simulink model "simple_FXTESO_ANSFT"  (R2024b)
settings: Solver=ode4  StartTime=0.0  StopTime=10  FixedStep=0.01  RelTol=1e-3
model workspace (MAT data in the model file):
  tra1 = [0 2 0 -2 0 2]
  tra2 = [0 2 2 2 2 0]
  tra3 = [0 0 2 2 2 2]
values from neighbouring files (symbols this model uses):
  F = 5    [assignment3.m]
undefined symbols (not defined in the file or in its folder): Light, MIL
libraries: dspobslib x7, simulink x3, robotcorelib x1, aerolibwind2 x1
settings Model: Creator=Adan Daniel  LastModifiedBy=danyy
settings OptimizationCC: ReuseModelBlockBuffer=off
settings RTWCC: GPUComputeCapability=3.5

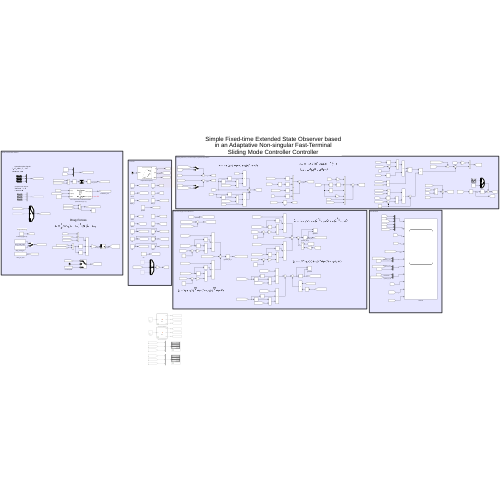
[thumbnail: Simulink's stored preview of the top-level diagram]
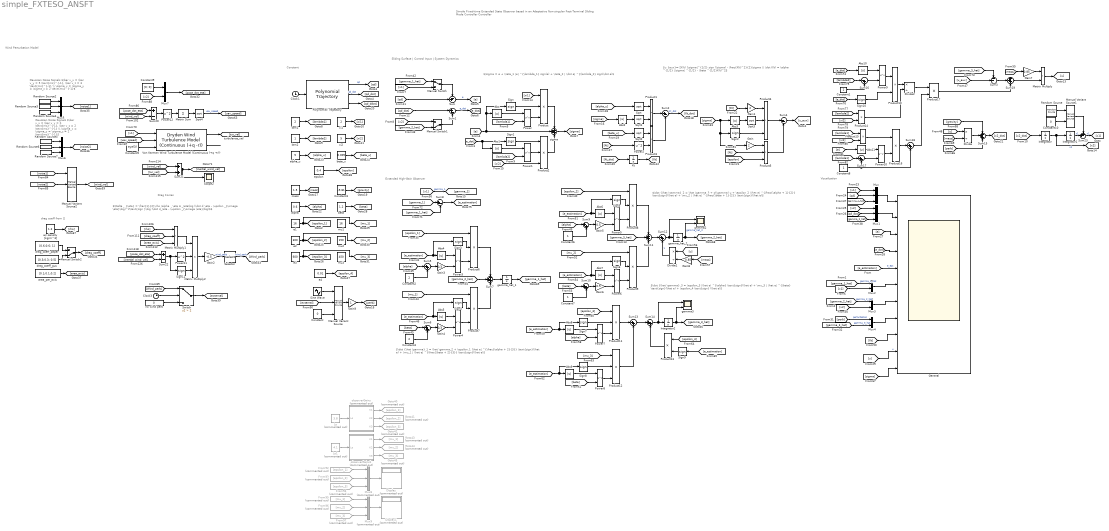
== system simple_FXTESO_ANSFT ==
  note: Extended High-Gain Observer
  note: Sliding Surface | Control Input | System Dynamics
  note: Constant
  note: Visualization
  note: Simple Fixed-time Extended State Observer based in an Adaptative Non-singular Fast-Terminal Sliding Mode Controller Controller
  note: $\dot {\hat \gamma}_1 = \hat \gamma_2 + \epsilon_1 |\hat e| ^{\frac{\alpha + 2}{3}} \text{sign}(\hat e) + \mu_1 | \hat e| ^{\frac{\beta + 2}{3}} \text{sign}(\hat e)$
  note: $\dot {\hat \gamma}_3 = \epsilon_3 |\hat e| ^{\alpha} \text{sign}(\hat e) + \mu_3 | \hat e| ^{\beta} \text{sign}(\hat e) + \epsilon_4 \text{sign} (\hat e)$
  note: $\dot {\hat \gamma}_2 = \hat \gamma_3 + g(\gamma) u + \epsilon_2 |\hat e| ^{\frac{\alpha + 1}{2}} \text{sign}(\hat e) + \mu_2 | \hat e| ^{\frac{\beta + 1}{2}} \text{sign}(\hat e)$
  note: $\sigma = e + \zeta_1 |e| ^{\lambda_1} sign(e) + \zeta_2 | \dot e| ^{\lambda_2} sign(\dot e)$
  note: $u_{aux}=-2K(t) |\sigma|^{1/2} sign (\sigma) - \frac{K(t)^2}{2}\sigma \\ \dot K(t) = \alpha ^{1/2} |\sigma| ^{1/2} - \beta ^{1/2}K(t)^2$
  note: Gaussian Noise Signals
      | $\bar v_x = \bar v_y = 6 \text{ms}^{-1}, \bar v_z = 2 \text{ms}^{-1} \\ \sigma_x = \sigma_y = \sigma_z = 2 \text{ms}^{-1}$
  note: $\Delta _ {\eta} = \frac{1}{2}\rho \alpha _ \eta A _\eta\big (\dot d_\eta - \upsilon _{\omega \eta}\big)^2\text{sign }\big (\dot d_\eta - \upsilon _{\omega \eta}\big)$$
  note: Gaussian Noise Signals
      | $\bar v_x = \bar v_y = 5 \text{ms}^{-1}, \bar v_z = 3 \text{ms}^{-1} \\ \sigma_x = \sigma_y = \sigma_z = 2 \text{ms}^{-1}$
  note: Wind Perturbation Model
  note: Drag Forces
  note: drag coeff from []
  Abs{,1..11} (12 alike) : Abs  SaturateOnIntegerOverflow=off
  Clock1 : Clock
  Clock3 : Clock
  Constant : Constant  Value=0
  Constant1 : Constant  Value=2
  Constant10 : Constant  Value=0
  Constant2 : Constant  Value=2
  Constant3 : Constant  Value=-9.81
  Constant4 : Constant  Value=2
  Constant5 : Constant  Value=eye(3)
  Constant6 : Constant
  Constant7 : Constant
  Constant8 : Constant
  Constant9 : Constant  Value=[0; 0]
  Display : Display  Commented=on
  Display1 : Display  Commented=on
  Divide : Product  Inputs=*/
  Divide1 : Product  Inputs=*/
  Divide2 : Product  Inputs=*/
  From92 : From  Commented=on  GotoTag=epsilon_1
  From93 : From  Commented=on  GotoTag=epsilon_2
  From94 : From  Commented=on  GotoTag=epsilon_3
  From95 : From  Commented=on  GotoTag=mu_1
  From96 : From  Commented=on  GotoTag=mu_2
  From97 : From  Commented=on  GotoTag=mu_3
  Gain : Gain  Gain=2
  Gain1 : Gain  Gain=2
  Gain2 : Gain  Gain=-0.5
  Gain3 : Gain  Gain=1/3
  Gain4 : Gain  Gain=1/3
  Gain5 : Gain  Gain=0.5
  Gain6 : Gain  Gain=0.5
  Gain7 : Gain  Gain=0.85
  Gain8 : Gain  Gain=0.85
  Gain9 : Gain
  General : Scope  NumInputPorts=11
  Goto40 : Goto  Commented=on  GotoTag=epsilon_1
  Goto41 : Goto  Commented=on  GotoTag=epsilon_2
  Goto42 : Goto  Commented=on  GotoTag=epsilon_3
  Goto43 : Goto  Commented=on  GotoTag=mu_1
  Goto44 : Goto  Commented=on  GotoTag=mu_2
  Goto45 : Goto  Commented=on  GotoTag=mu_3
  Integrator : Integrator
  Integrator1 : Integrator  InitialCondition=0.1
  Integrator2 : Integrator  InitialCondition=-9.81
  Kt : Integrator
  Lo : Constant  Commented=on  Value=3.8
  Lo1 : Constant  Commented=on  Value=4.1
  Manual Variant Source : simulink/Signal Routing/Manual Variant Source  NumChoices=3  LabelModeActiveChoice=V_2
  Manual Variant Source1 : simulink/Signal Routing/Manual Variant Source  NumChoices=2  LabelModeActiveChoice=V_2
  Manual Variant Source2 : simulink/Signal Routing/Manual Variant Source  NumChoices=3  LabelModeActiveChoice=V_1
  Manual Switch : ManualSwitch
  Manual Switch1 : ManualSwitch  CurrentSetting=0
  Manual Switch2 : ManualSwitch  CurrentSetting=0
  Matrix Sum : Sum  Inputs=+
  Matrix Multiply : Product
  Matrix Multiply1 : Product  Inputs=3
  Matrix Multiply2 : Product  Inputs=3
  Mux{,1,5..6} (4 alike) : Mux  Inputs=3
  Mux{2..4,7} (4 alike) : Mux  Inputs=2
  Mux8 : Mux  Commented=on  Inputs=3
  Mux9 : Mux  Commented=on  Inputs=3
  Polynomial Trajectory : robotcorelib/Polynomial Trajectory  WaypointSource=Internal  Waypoints=[0 0 -1 1 -1 1 -1 1 -1 1]/5  TimePoints=[0 1 2 3 4 5 6 7 8 9]  TimeInterval=[ 1, 4 ]  Method=Cubic Polynomial  ParameterSource=Internal  VelocityBoundaryCondition=zeros( 1, 10)  AccelerationBoundaryCondition=zeros( 2, 5 )  SimulateUsing=Interpreted execution
  Power{,1,3..10} (10 alike) : Math  Operator=pow
  Power11 : Math  Operator=square
  Power12 : Math  Operator=square
  Power2 : Math  Operator=square
  Product{,2,4..9,11..12} (10 alike) : Product  Inputs=3
  Product{1,3,10,13..17} (8 alike) : Product
  Random Source : dspobslib/Random Source  SrcType=Gaussian  NormMethod=Ziggurat  CltLength=12  MinVal=0  MaxVal=1  MeanVal=0.001  VarVal=0.001 * 0.001  RepMode=Not repeatable  rawSeed=1  IsInherit=off  SampMode=Discrete  SampTime=0.01  SampFrame=1  DataType=Double  OutComplex=Real  OutputFrames=off
  Random Source2 : dspobslib/Random Source  SrcType=Gaussian  NormMethod=Ziggurat  CltLength=12  MinVal=0  MaxVal=1  MeanVal=5  VarVal=2  RepMode=Not repeatable  rawSeed=1  IsInherit=off  SampMode=Discrete  SampTime=1  SampFrame=1  DataType=Double  OutComplex=Real  OutputFrames=off
  Random Source3 : dspobslib/Random Source  SrcType=Gaussian  NormMethod=Ziggurat  CltLength=12  MinVal=0  MaxVal=1  MeanVal=5  VarVal=2  RepMode=Not repeatable  rawSeed=1  IsInherit=off  SampMode=Discrete  SampTime=1  SampFrame=1  DataType=Double  OutComplex=Real  OutputFrames=off
  Random Source4 : dspobslib/Random Source  SrcType=Gaussian  NormMethod=Ziggurat  CltLength=12  MinVal=0  MaxVal=1  MeanVal=3  VarVal=2  RepMode=Not repeatable  rawSeed=1  IsInherit=off  SampMode=Discrete  SampTime=1  SampFrame=1  DataType=Double  OutComplex=Real  OutputFrames=off
  Random Source5 : dspobslib/Random Source  SrcType=Gaussian  NormMethod=Ziggurat  CltLength=12  MinVal=0  MaxVal=1  MeanVal=6  VarVal=2  RepMode=Not repeatable  rawSeed=1  IsInherit=off  SampMode=Discrete  SampTime=1  SampFrame=1  DataType=Double  OutComplex=Real  OutputFrames=off
  Random Source6 : dspobslib/Random Source  SrcType=Gaussian  NormMethod=Ziggurat  CltLength=12  MinVal=0  MaxVal=1  MeanVal=6  VarVal=2  RepMode=Not repeatable  rawSeed=1  IsInherit=off  SampMode=Discrete  SampTime=1  SampFrame=1  DataType=Double  OutComplex=Real  OutputFrames=off
  Random Source7 : dspobslib/Random Source  SrcType=Gaussian  NormMethod=Ziggurat  CltLength=12  MinVal=0  MaxVal=1  MeanVal=2  VarVal=2  RepMode=Not repeatable  rawSeed=1  IsInherit=off  SampMode=Discrete  SampTime=1  SampFrame=1  DataType=Double  OutComplex=Real  OutputFrames=off
  Scope2 : Scope
  Selector : Selector  InputPortWidth=3  IndexOptions=Index vector (dialog)  Indices=[3]  OutputSizes=1
  Sign{,1..11} (12 alike) : Signum
  Sine Wave : Sin  Amplitude=0.45  Frequency=0.25  SampleTime=0
  Sqrt{,1..4} (5 alike) : Sqrt
  Sum : Sum  Inputs=-+|
  Sum{1..2,8,17} (4 alike) : Sum  Inputs=|+-
  Sum{5..6,9..10,12..14,18} (8 alike) : Sum  Inputs=|++
  Sum{7,11,15,19} (4 alike) : Sum  Inputs=+++
  Sum16 : Sum  Inputs=|-+
  Sum20 : Sum  Inputs=+-
  Sum21 : Sum
  Sum22 : Sum  Inputs=+-
  Sum23 : Sum  Inputs=++|
  Sum3 : Sum  Inputs=--|
  Sum4 : Sum  Inputs=|--
  Switch : Switch  Criteria=u2 > Threshold  Threshold=2  SaturateOnIntegerOverflow=off  InputSameDT=off
  Von Karman Wind Turbulence Model (Continuous (+q +r)) : aerolibwind2/Dryden Wind Turbulence Model  (Continuous (+q -r))  units=Metric (MKS)  spec=MIL-F-8785C  model=Continuous Von Karman (+q +r)  W20=15  Wdeg=0  TurbProb=10^-2 - Light  L_high=762  Wingspan=10  ts=0.1  Seed=[23341 23342 23343 23344]  T_on=on
      settings: LibrarySourceBlock=|
      | aerolibwind2/Von Karman Wind Turbulence Model
      | (Continuous (+q +r))
  air density [kg/m^3] : Constant  Value=1.2
  alpha : Constant  Value=0.6
  alpha_u : Constant  Value=5
  area_per_axis : Constant  Value=[0.1;0.1;0.2]
  beta : Constant  Value=1.2
  beta_u : Constant  Value=0.005
  drag_coeff_gus : Constant  Value=[0.3;0.3; 0.5]
  drag_coeff_paper : Constant  Value=[0.6;0.6; 1]
  e1 : Constant  Value=16
  e2 : Constant  Value=300
  e3 : Constant  Value=600
  e4 : Constant  Value=0.01
  epsilon : Constant  Value=0.4
  gamma2 : Scope  NumInputPorts=2
  gamma3 : Scope  NumInputPorts=2
  gamma_hat_1 : Integrator
  gamma_hat_2 : Integrator
  lam1 : Constant  Value=2
  lam2 : Constant
  mass : Constant  Value=1.5
  mu1 : Constant  Value=16
  mu2 : Constant  Value=150
  mu3 : Constant  Value=450
  no wind perb : Constant  Value=0
  observerGains : MATLAB Function  Commented=on  TreatAsAtomicUnit=on
  observerGains1 : MATLAB Function  Commented=on  TreatAsAtomicUnit=on
  sigma : Sum  Inputs=+++
  xi1 : Constant  Value=2
  xi2 : Constant  Value=5
  wires:
  Integrator1/1 -> Sum23/2  "x1"
  Integrator/1 -> [x2], Integrator1/1  "x2"
  Sum1/1 -> [e_dot]  "e_dot"
  Mux/1 -> General/1
  [x2_dot] -> Integrator/1
  Clock1/1 -> Polynomial Trajectory/1
  Polynomial Trajectory/3 -> [qd_ddot]
  gamma_hat_1/1 -> [gamma_1_hat]
  [gamma_1] -> Sum8/1
  [gamma_1_hat] -> Sum8/2
  Sum8/1 -> [e_estimation]
  gamma_hat_2/1 -> gamma2/2, [gamma_2_hat]  "gamma_hat_2"
  [e_estimation] -> General/5  "e_est"
  [gamma_1_hat] -> Mux2/1  "gamma_1_hat"
  [gamma_2_hat] -> Mux3/1  "gamma_2_hat"
  Mux2/1 -> General/6
  [x1] -> Mux2/2
  Mux3/1 -> General/7
  [x1] -> Manual Switch/2
  [x2] -> Manual Switch1/1
  [qd] -> Mux/2
  Polynomial Trajectory/1 -> [qd]  "qd"
  Polynomial Trajectory/2 -> [qd_dot]  "qd_dot"
  [qd] -> Sum/2
  [qd_dot] -> Sum1/1
  Sum/1 -> [e]  "e"
  lam1/1 -> [lambda1]
  lam2/1 -> [lambda2]
  xi1/1 -> [xi1]
  xi2/1 -> [xi2]
  [x1] -> Mux/1
  [qd_dot] -> Mux1/2
  [x2] -> Mux1/1
  Mux1/1 -> General/2
  [e] -> General/3
  [e_dot] -> General/4
  [x1] -> [gamma_1]  "gamma_1"
  [x2] -> Mux3/2
  [perb] -> Mux4/1  "perturbation"
  Manual Variant Source/1 -> Gain9/1
  Sine Wave/1 -> Manual Variant Source/1
  Mux4/1 -> General/8
  [gamma_3_hat] -> Mux4/2  "gamma_3_hat"
  mass/1 -> [mass]
  [gamma_1_hat] -> Mux/3
  [gamma_2_hat] -> Mux1/3
  Constant/1 -> Manual Variant Source/3
  Manual Switch/1 -> Sum/1
  Manual Switch1/1 -> Sum1/2
  [gamma_2_hat] -> Manual Switch1/2
  [gamma_1_hat] -> Manual Switch/1
  Constant3/1 -> [gravity]
  [Kt] -> General/9
  alpha/1 -> [alpha]
  [u] -> General/10  "u"
  [u] -> Divide/1
  [e] -> sigma/2, Abs/1, Sign/1
  Abs/1 -> Power/1
  [lambda1] -> Power/2
  Power/1 -> Product/3
  Sign/1 -> Product/2
  sigma/1 -> [sigma]
  Power1/1 -> Product2/2
  [e_dot] -> Abs1/1, Sign1/1
  [lambda2] -> Power1/2
  Abs1/1 -> Power1/1
  Sign1/1 -> Product2/1
  Product2/1 -> sigma/3
  Product/1 -> sigma/1
  [xi1] -> Product/1
  [xi2] -> Product2/3
  beta_u/1 -> [beta_u]
  alpha_u/1 -> [alpha_u]
  [Kt] -> Power2/1
  [alpha_u] -> Sqrt/1
  [sigma] -> Abs2/1
  Abs2/1 -> Sqrt1/1
  Sqrt1/1 -> Product1/2
  Power2/1 -> Product3/2
  [beta_u] -> Sqrt2/1
  Sqrt/1 -> Product1/1
  Product3/1 -> Sum2/2
  Product1/1 -> Sum2/1
  Sqrt2/1 -> Product3/1
  Sum2/1 -> [Kt_dot]  "Kt_dot"
  [Kt_dot] -> Kt/1
  Kt/1 -> [Kt]
  Sum4/1 -> [u_aux]
  e1/1 -> [mu_1], [epsilon_1]
  e2/1 -> [mu_2], [epsilon_2]
  e4/1 -> [epsilon_4]
  e3/1 -> [mu_3], [epsilon_3]
  beta/1 -> [beta]
  [e_estimation] -> Sign3/1, Abs4/1
  Abs4/1 -> Power3/1
  Power3/1 -> Product6/3
  Sign3/1 -> Product6/2
  [epsilon_1] -> Product6/1
  [alpha] -> Sum5/1
  Constant2/1 -> Sum5/2
  Sum5/1 -> Gain3/1
  Gain3/1 -> Power3/2
  Abs5/1 -> Power4/1
  [beta] -> Sum6/1
  Power4/1 -> Product7/3
  Sign4/1 -> Product7/2
  Sum6/1 -> Gain4/1
  Gain4/1 -> Power4/2
  [mu_1] -> Product7/1
  Constant4/1 -> Sum6/2
  [e_estimation] -> Sign4/1, Abs5/1
  [gamma_2_hat] -> Sum7/2
  Product7/1 -> Sum7/3
  Product6/1 -> Sum7/1
  Sum7/1 -> gamma_hat_1/1
  Power6/1 -> Product9/3
  [gamma_3_hat] -> Sum11/2
  Power5/1 -> Product8/3
  Product9/1 -> Sum11/3
  [e_estimation] -> Sign5/1, Abs6/1
  [mu_2] -> Product9/1
  Gain6/1 -> Power6/2
  Sign5/1 -> Product8/2
  [e_estimation] -> Sign6/1, Abs7/1
  [alpha] -> Sum9/1
  [beta] -> Sum10/1
  Sum9/1 -> Gain5/1
  Abs6/1 -> Power5/1
  Abs7/1 -> Power6/1
  Sum10/1 -> Gain6/1
  Constant7/1 -> Sum10/2
  Sign6/1 -> Product9/2
  Gain5/1 -> Power5/2
  [epsilon_2] -> Product8/1
  Constant6/1 -> Sum9/2
  Product8/1 -> Sum11/1
  Matrix Multiply/1 -> [u]
  [u] -> Divide1/1
  [mass] -> Gain8/1
  Sum12/1 -> gamma2/1, gamma_hat_2/1
  Sum11/1 -> Sum12/1
  Divide1/1 -> Sum12/2  "u"
  Sign7/1 -> Product11/2
  Abs8/1 -> Power7/1
  [e_estimation] -> Abs8/1, Sign7/1
  [alpha] -> Power7/2
  Power7/1 -> Product11/3
  [epsilon_3] -> Product11/1
  [mu_3] -> Product12/1
  [e_estimation] -> Abs9/1, Sign8/1
  [beta] -> Power8/2
  Abs9/1 -> Power8/1
  Power8/1 -> Product12/3
  Sign8/1 -> Product12/2
  Product11/1 -> Sum13/1
  Product12/1 -> Sum13/2
  [e_estimation] -> Sign9/1
  [epsilon_4] -> Product13/1
  Sign9/1 -> Product13/2
  Sum13/1 -> Sum14/1
  Product13/1 -> Sum14/2
  Sum14/1 -> gamma3/1, Integrator2/1
  Integrator2/1 -> gamma3/2, [gamma_3_hat]
  Sum15/1 -> [x2_dot]
  [sigma] -> General/11
  [external] -> Manual Variant Source/2
  [mass] -> Divide/2
  Divide/1 -> Sum15/2
  [perb] -> Sum15/3
  [gravity] -> Sum15/1
  [mass] -> Gain7/1
  [u_aux] -> Sum3/2
  [gamma_3_hat] -> Sum3/1
  [e_dot] -> Abs10/1
  Sum16/1 -> Power9/2
  Sign10/1 -> Product10/2
  Abs10/1 -> Power9/1
  Product14/1 -> Divide2/2
  Constant1/1 -> Sum16/2
  [lambda2] -> Sum16/1
  Power9/1 -> Product10/1
  [lambda2] -> Product14/1
  [e_dot] -> Sign10/1
  Product10/1 -> Divide2/1
  [xi2] -> Product14/2
  Product15/1 -> Product16/1
  Product16/1 -> Sum18/1
  Power10/1 -> Product16/2
  Constant8/1 -> Sum18/2, Sum17/2
  [xi1] -> Product15/2
  [lambda1] -> Product15/1
  Abs11/1 -> Power10/1
  [lambda1] -> Sum17/1
  [e] -> Abs11/1
  Sum17/1 -> Power10/2
  Divide2/1 -> Product17/1
  Sum18/1 -> Product17/2
  Sum19/1 -> Matrix Multiply/2
  Sum3/1 -> Sum19/2
  Product17/1 -> Sum19/3
  drag_coeff_gus/1 -> Manual Switch2/2
  Mux6/1 -> [noise2]
  [area_axis] -> Matrix Multiply1/3
  [x2] -> Mux7/2
  [x1] -> Von Karman Wind Turbulence Model (Continuous (+q +r))/1
  Random Source5/1 -> Mux6/1
  [pose_dot_eta] -> Sum22/1
  Gain2/1 -> Selector/1  "wind_perb"
  no wind perb/1 -> Switch/3
  [noise1] -> Manual Variant Source2/1
  [uav_speed] -> Von Karman Wind Turbulence Model (Continuous (+q +r))/2
  Manual Variant Source2/1 -> [wind_vel]
  Sqrt4/1 -> [uav_speed]  "uav_speed"
  [drag_coeff] -> Matrix Multiply1/2
  Von Karman Wind Turbulence Model (Continuous (+q +r))/1 -> [tur_vel]
  [inertial_wind_vel] -> Sum22/2
  Constant9/1 -> Mux7/1
  Matrix Multiply2/1 -> Gain2/1
  air density [kg/m^3]/1 -> [rho]
  Manual Switch2/1 -> [drag_coeff]
  Sum22/1 -> Sign11/1, Power11/1
  Random Source3/1 -> Mux5/2
  Random Source7/1 -> Mux6/3
  Sum21/1 -> Scope2/1, [inertial_wind_vel]
  [rho] -> Matrix Multiply1/1
  Switch/1 -> [external]
  [pose_dot_eta] -> Sum20/1
  Mux7/1 -> [pose_dot_eta]
  area_per_axis/1 -> [area_axis]
  [wind_vel] -> Sum21/1
  Power12/1 -> Matrix Sum/1
  Selector/1 -> [Wind_perb]  "wind_perb"
  Matrix Multiply1/1 -> Matrix Multiply2/1
  Sum20/1 -> Power12/1
  drag_coeff_paper/1 -> Manual Switch2/1
  Von Karman Wind Turbulence Model (Continuous (+q +r))/2 -> ?
  Random Source4/1 -> Mux5/3
  Power11/1 -> Matrix Multiply2/2
  Clock3/1 -> Switch/2
  Random Source2/1 -> Mux5/1
  Mux5/1 -> [noise1]
  [tur_vel] -> Sum21/2
  [noise2] -> Manual Variant Source2/2
  Constant5/1 -> Von Karman Wind Turbulence Model (Continuous (+q +r))/3
  [wind_vel] -> Sum20/2
  [Wind_perb] -> Switch/1
  Matrix Sum/1 -> Sqrt4/1
  Sign11/1 -> Matrix Multiply2/3
  Random Source6/1 -> Mux6/2
  Sum23/1 -> [x1]  "x1"
  Manual Variant Source1/1 -> Sum23/1
  Random Source/1 -> Manual Variant Source1/1
  Constant10/1 -> Manual Variant Source1/2
  Product4/1 -> Sum4/1
  Abs3/1 -> Sqrt3/1
  Sign2/1 -> Product4/3
  [Kt] -> Gain1/1
  [epsilon] -> Product5/3
  Product5/1 -> Sum4/2
  Gain1/1 -> Product4/1
  Sqrt3/1 -> Product4/2
  [sigma] -> Abs3/1, Gain/1, Sign2/1
  [Kt] -> Product5/2
  Gain/1 -> Product5/1
  epsilon/1 -> [epsilon]
  Lo/1 -> observerGains/1(Lo)
  observerGains/1(K1) -> Goto40/1
  observerGains/2(K2) -> Goto41/1
  observerGains/3(K3) -> Goto42/1
  From94/1 -> Mux8/3
  From93/1 -> Mux8/2
  From92/1 -> Mux8/1
  Mux8/1 -> Display/1
  observerGains1/2(K2) -> Goto44/1
  observerGains1/3(K3) -> Goto45/1
  Lo1/1 -> observerGains1/1(Lo)
  observerGains1/1(K1) -> Goto43/1
  From95/1 -> Mux9/1
  From96/1 -> Mux9/2
  Mux9/1 -> Display1/1
  From97/1 -> Mux9/3
  Gain7/1 -> Matrix Multiply/1
  Gain8/1 -> Divide1/2
  Gain9/1 -> [perb]

== matlab function simple_FXTESO_ANSFT/observerGains ==
  data: Lo input; K1 output; K2 output; K3 output
function [K1, K2, K3] = fcn(Lo)

K1 = 3 * Lo ^ (5/3);

K2 = 2 * Lo ^ (10/3);

K3 = (4/9) * Lo ^ (5);

== matlab function simple_FXTESO_ANSFT/observerGains1 ==
  data: Lo input; K1 output; K2 output; K3 output
function [K1, K2, K3] = fcn(Lo)

K1 = 3 * Lo ^ (5/3);

K2 = 2 * Lo ^ (10/3);

K3 = (4/9) * Lo ^ (5);
